simulink model "odev6_iremelmas_kara"  (R2023b)
settings: Solver=ode23tb  StartTime=0.0  StopTime=5  MaxStep=0.00001  RelTol=1e-5  EnableMultiTasking=on
libraries: spsSeriesRLCBranchLib x17, spsDiodeLib x2, spsThyristorLib x2, spsVoltageMeasurementLib x2, spsDCVoltageSourceLib x1, spsACVoltageSourceLib x1, powerlib_extras x1, spsCurrentMeasurementLib x1, spsDCMachineLib x1, spsFourierLib x1, spsMeanLib x1, spsRMSLib x1
settings Model: Creator=bb  LastModifiedBy=ireme
settings SolverCC: AlgebraicLoopSolver=TrustRegion
settings DataIOCC: SaveFormat=Array  SignalLoggingSaveFormat=ModelDataLogs  SaveOutput=off  SignalLogging=off  SaveTime=off  ReturnWorkspaceOutputs=off
settings OptimizationCC: ExpressionDepthLimit=2147483647  InitFltsAndDblsToZero=on  LifeSpan=inf
settings DebuggingCC: SaveWithParameterizedLinksMsg=none  UnderspecifiedInitializationDetection=Classic  MergeDetectMultiDrivingBlocksExec=none  SignalResolutionControl=TryResolveAllWithWarning  SolverPrmCheckMsg=warning  FcnCallInpInsideContextMsg=warning  UnconnectedInputMsg=warning  UnconnectedOutputMsg=warning  UnconnectedLineMsg=warning  StateNameClashWarn=warning  SFUnexpectedBacktrackingDiag=warning  SFNoUnconditionalDefaultTransitionDiag=warning  SFExecutionAtInitializationDiag=none  ArithmeticOperatorsInVariantConditions=warning
settings HardwareCC: ProdBitPerPointer=32  ProdBitPerSizeT=32  ProdBitPerPtrDiffT=32  ProdLargestAtomicFloat=None  ProdIntDivRoundTo=Undefined  ProdEndianess=Unspecified  ProdWordSize=32  ProdHWDeviceType=32-bit Generic
settings ModelReferenceCC: EnableRefExpFcnMdlSchedulingChecks=on  PropagateSignalLabelsOutOfModel=off
settings SFSimCC: SimUseLocalCustomCode=off  CustomCodeUndefinedFunction=UseInterfaceOnly
settings RTWCC: RTWUseLocalCustomCode=off
settings CodeAppCC: StateflowObjectComments=on
settings GRTTargetCC: TargetFcnLib=ansi_tfl_tmw.mat  TargetLangStandard=C89/C90 (ANSI)  CombineOutputUpdateFcns=off  GRTInterface=on
settings ConfigComp: CovMetricSettings=dw  CovSaveCumulativeToWorkspaceVar=on  CovSaveSingleToWorkspaceVar=on  CovExternalEMLEnable=off
settings SimscapeCC: SimscapeNormalizeSystem=off

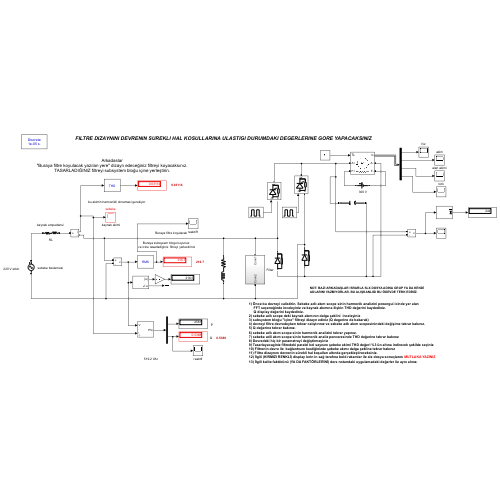
[thumbnail: Simulink's stored preview of the top-level diagram]
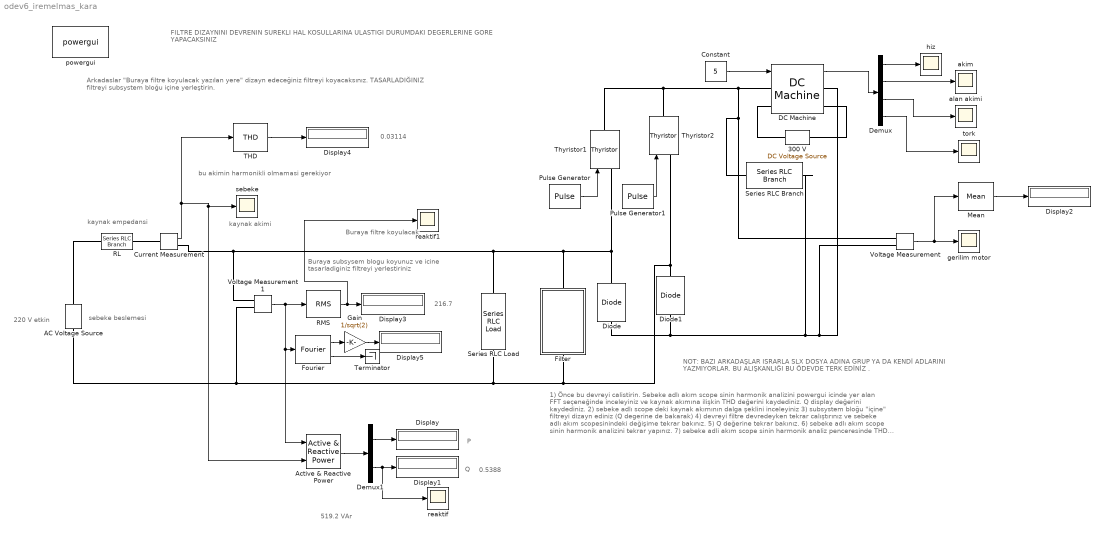
== system odev6_iremelmas_kara ==
  note: 220 V etkin
  note: NOT: BAZI ARKADAŞLAR ISRARLA SLX DOSYA ADINA GRUP YA DA KENDİ ADLARINI YAZMIYORLAR. BU ALIŞKANLIĞI BU ÖDEVDE TERK EDİNİZ .
  note: 216.7
  note: 0.5388
  note: 0.03114
  note: 519.2 VAr
  note: Q
  note: P
  note: Buraya filtre koyulacak
  note: Arkadaslar
      | "Buraya filtre koyulacak yazılan yere" dizayn edeceğiniz filtreyi koyacaksınız.
      | TASARLADIĞINIZ filtreyi subsystem bloğu içine yerleştirin.
  note: kaynak empedansi
  note: 1) Önce bu devreyi calistirin. Sebeke adlı akım scope sinin harmonik analizini powergui icinde yer alan
      | FFT seçeneğinde inceleyiniz ve kaynak akımına ilişkin THD değerini kaydediniz.
      | Q display değerini kaydediniz.
      | 2) sebeke adlı scope deki kaynak akımının dalga şeklini inceleyiniz
      | 3) subsystem bloğu "içine" filtreyi dizayn ediniz (Q degerine de bakarak)
      | 4) devreyi filtre devredeyken tekrar calıştırınız ve sebeke adlı akım scopesinindeki değişime tekrar bakınız.
      | 5) Q değerine tekrar bakınız.
      | 6) sebeke adlı akım scope sinin harmonik analizini tekrar yapınız.
      | 7) sebeke adli akım scope sinin harmonik analiz penceresinde THD değerine tekrar bakınız
      | 8) Devredeki hiç bir parametreyi değiştirmeyiniz
      | 9) Tasarlayacaginiz filtredeki paralel kol sayısını şebeke akimi THD değeri %3 ün altına indirecek şekilde seçiniz
      | 10) Filtrenin devre ile bağlantısını kestiğinizde şebeke akımı dalga şekline tekrar bakınız
      | 11) Filtre dizaynını devrenin sürekli hal koşulları altında gerçekleştireceksiniz.
      | 12) İlgili (KIRMIZI RENKLİ) display lerin in sağ tarafına bold rakamlar ile slx dosya sonuçlarını MUTLAKA YAZINIZ
      | 13) İlgili kalite faktörünü (YA DA FAKTÖRLERİNİ) ders notundaki uygulamadaki değerler ile aynı alınız.
  note: kaynak akimi
  note: bu akimin harmonikli olmamasi gerekiyor
  note: Buraya subsysem blogu koyunuz
      | ve icine tasarladiginiz  filtreyi yerlestiriniz
  note: sebeke beslemesi
  note: FILTRE DIZAYNINI DEVRENIN SUREKLI HAL KOSULLARINA ULASTIGI DURUMDAKI DEGERLERINE GORE YAPACAKSINIZ
  " 300 V" : spsDCVoltageSourceLib/DC Voltage Source  Amplitude=300  Measurements=None
  AC Voltage Source : spsACVoltageSourceLib/AC Voltage Source  Amplitude=220*sqrt(2)  Phase=0  Frequency=50  SampleTime=0  Measurements=None  BusType=swing  Pref=10e3  Qref=0  Qmin=-inf  Qmax=+inf
  Active & Reactive Power : powerlib_extras/Measurements/Active & Reactive Power  f1=50
  Constant : Constant  Value=5
  Current Measurement : spsCurrentMeasurementLib/Current Measurement  PhasorSimulation=off  OutputType=Complex  PSBequivalent=0
  DC Machine : spsDCMachineLib/DC Machine  PresetModel=01: 5HP 240V 1750RPM Field:300V  MechanicalLoad=Torque TL  FieldType=Wound  ShowDetailedParameters=on  MeasurementBus=off  RLa=[2.581 0.028]  RLf=[281.2 156]  Laf=0.9483  MachineConstant=Torque constant (N.m/A)  Ke=1.8  Kt=1.8  J=0.02215  Bm=0.002953  Tf=0.5161  w0=0  Ifinit=1.06685632871799  TsPowergui=0  TsBlock=-1
  Demux : Demux
  Demux1 : Demux  Outputs=2
  Diode : spsDiodeLib/Diode  Ron=0.001  Lon=0  Vf=0.8  IC=0  UseSnubber=off  Rs=500  Cs=250e-9  Measurements=off
  Diode1 : spsDiodeLib/Diode  Ron=0.001  Lon=0  Vf=0.8  IC=0  UseSnubber=off  Rs=500  Cs=250e-9  Measurements=off
  Display{,1..5} (6 alike) : Display
  Filter : Subsystem
  Fourier : spsFourierLib/Fourier  Freq=50  n=1  InInit=[0, 0]  Ts=0
  Gain : Gain  Gain=1/sqrt(2)
  Mean : spsMeanLib/Mean  Freq=50  Vinit=0  Ts=0
  Pulse Generator : DiscretePulseGenerator  PulseType=Time based  Period=0.02  PulseWidth=15  PhaseDelay=0.66*0.01
  Pulse Generator1 : DiscretePulseGenerator  PulseType=Time based  Period=0.02  PulseWidth=15  PhaseDelay=0.66*0.01+0.01
  RL : spsSeriesRLCBranchLib/Series RLC Branch  LConnTagsString=__new0  RConnTagsString=__new0  BranchType=RL  Resistance=0.2  Inductance=6e-3  SetiL0=off  InitialCurrent=0  Capacitance=1e-6  Setx0=off  InitialVoltage=0  Measurements=None
  RMS : spsRMSLib/RMS  TrueRMS=on  Freq=50  RMSInit=100  Ts=0
  Series RLC Branch : spsSeriesRLCBranchLib/Series RLC Branch  LConnTagsString=__new0  RConnTagsString=__new0  BranchType=C  Resistance=1  Inductance=1e-3  SetiL0=off  InitialCurrent=0  Capacitance=2e-1  Setx0=off  InitialVoltage=0  Measurements=None
  Series RLC Load : spsSeriesRLCLoadLib/Series RLC Load  LConnTagsString=a  RConnTagsString=__new0  NominalVoltage=220  NominalFrequency=50  ActivePower=10e2  InductivePower=10000  CapacitivePower=0  Setx0=off  InitialVoltage=0  SetiL0=off  InitialCurrent=0  Measurements=None  LoadType=constant Z
  THD : spsTHDLib/THD  Freq=50  Ts=0
  Terminator : Terminator
  Thyristor1 : spsThyristorLib/Thyristor  Ron=1e-3  Lon=0  Vf=0.8  IC=0  Rs=200  Cs=4e-6  Measurements=off
      settings: AttributesFormatString=\n
  Thyristor2 : spsThyristorLib/Thyristor  Ron=1e-3  Lon=0  Vf=0.8  IC=0  Rs=200  Cs=4e-6  Measurements=off
      settings: AttributesFormatString=\n
  Voltage Measurement : spsVoltageMeasurementLib/Voltage Measurement  PhasorSimulation=off  OutputType=Complex  PSBequivalent=0
  Voltage Measurement1 : spsVoltageMeasurementLib/Voltage Measurement  PhasorSimulation=off  OutputType=Complex  PSBequivalent=0
  akim : Scope
  alan akimi : Scope
  gerilim motor : Scope
  hiz : Scope
  powergui : spspowerguiLib/powergui  SimulationMode=Discrete  SampleTime=1e-5  frequency=50  Iterations=50  frequencyindice=0  Pbase=100e6  ErrMax=1e-4  UnitsV=kV  UnitsW=MW  buscounter=0  FunctionMessages=off  echomessages=off  EnableUseOfTLC=off  CurrentSourceSwitches=off  DisableSnubberDevices=off  DisableRonSwitches=off  DisableVfSwitches=off  DisplayEquations=off  AutomaticDiscreteSolvers=off  SolverType=Tustin  Interpol=off  ExternalGateDelay=off  methode=off  Ts=0  x0status=steady  SPID=off  SwTol=0  HookPort=off  NonlinearTolerance=1e-4  nMaxIteration=100  ContinueOnMaxIteration=off  RestoreLinks=warning  ResistiveCurrentMeasurement=off  Frange=[0:2:500]  Ylog=off  Xlog=on  ShowGrid=off  save=off  variable=ZData  structure=sebeke  ZoomFFT=off  StartTime=1.6  cycles=4  DisplayStyle=4  fundamental=50  FreqAxis=off  MaxFrequency=1000  frequencyindicesteady=1  RmsSteady=1  display=off
  reaktif : Scope
  reaktif1 : Scope
  sebeke : Scope
  tork : Scope
  wires:
  Constant/1 -> DC Machine/1
  DC Machine/1 -> Demux/1
  Demux/1 -> hiz/1
  Demux/2 -> akim/1
  Demux/3 -> alan akimi/1
  Demux/4 -> tork/1
  Current Measurement/1 -> THD/1, Active & Reactive Power/2, sebeke/1
  Voltage Measurement1/1 -> RMS/1, Fourier/1, Active & Reactive Power/1
  Active & Reactive Power/1 -> Demux1/1
  Demux1/1 -> Display/1
  Demux1/2 -> Display1/1, reaktif/1
  Voltage Measurement/1 -> Mean/1, gerilim motor/1
  Mean/1 -> Display2/1
  RMS/1 -> reaktif1/1, Display3/1
  THD/1 -> Display4/1
  Fourier/2 -> Terminator/1
  Fourier/1 -> Gain/1
  Gain/1 -> Display5/1
  Pulse Generator1/1 -> Thyristor2/1
  Pulse Generator/1 -> Thyristor1/1
  connections:
  " 300 V"/RConn1 -- DC Machine/LConn2
  " 300 V"/LConn1 -- DC Machine/RConn2
  Series RLC Branch/LConn1 -- Voltage Measurement/LConn1 -- Thyristor2/RConn1 -- Thyristor1/RConn1 -- DC Machine/LConn1
  Current Measurement/RConn1 -- Series RLC Load/LConn1 -- Filter/RConn1 -- Diode/RConn1 -- Thyristor1/LConn1 -- Voltage Measurement1/LConn1
  AC Voltage Source/LConn1 -- Filter/LConn1 -- Thyristor2/LConn1 -- Diode1/RConn1 -- Series RLC Load/RConn1 -- Voltage Measurement1/LConn2
  DC Machine/RConn1 -- Voltage Measurement/LConn2 -- Series RLC Branch/RConn1 -- Diode/LConn1 -- Diode1/LConn1
  AC Voltage Source/RConn1 -- RL/LConn1
  RL/RConn1 -- Current Measurement/LConn1

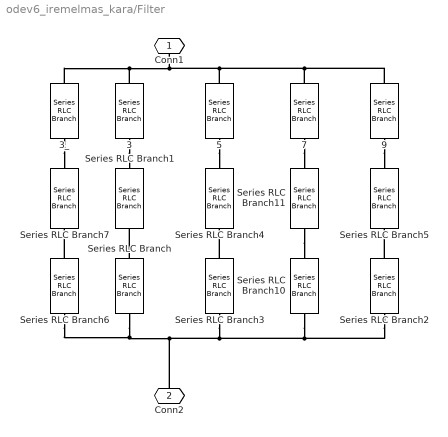
== system odev6_iremelmas_kara/Filter ==
  {3,5,7,9} (4 alike) : spsSeriesRLCBranchLib/Series RLC Branch  LConnTagsString=__new0  RConnTagsString=__new0  BranchType=C  Resistance=1  Inductance=1e-3  SetiL0=off  InitialCurrent=0  Capacitance=0.00013674  Setx0=off  InitialVoltage=0  Measurements=None
  3_ : spsSeriesRLCBranchLib/Series RLC Branch  LConnTagsString=__new0  RConnTagsString=__new0  BranchType=C  Resistance=1  Inductance=1e-3  SetiL0=off  InitialCurrent=0  Capacitance=0.00013674  Setx0=off  InitialVoltage=0  Measurements=None
  Series RLC Branch : spsSeriesRLCBranchLib/Series RLC Branch  LConnTagsString=__new0  RConnTagsString=__new0  BranchType=R  Resistance=0.2217  Inductance=1e-3  SetiL0=off  InitialCurrent=0  Capacitance=1e-6  Setx0=off  InitialVoltage=0  Measurements=None
  Series RLC Branch1 : spsSeriesRLCBranchLib/Series RLC Branch  LConnTagsString=__new0  RConnTagsString=__new0  BranchType=L  Resistance=1  Inductance=0.0082332  SetiL0=off  InitialCurrent=0  Capacitance=1e-6  Setx0=off  InitialVoltage=0  Measurements=None
  Series RLC Branch10 : spsSeriesRLCBranchLib/Series RLC Branch  LConnTagsString=__new0  RConnTagsString=__new0  BranchType=R  Resistance=0.095016  Inductance=1e-3  SetiL0=off  InitialCurrent=0  Capacitance=1e-6  Setx0=off  InitialVoltage=0  Measurements=None
  Series RLC Branch11 : spsSeriesRLCBranchLib/Series RLC Branch  LConnTagsString=__new0  RConnTagsString=__new0  BranchType=L  Resistance=1  Inductance=0.0015122  SetiL0=off  InitialCurrent=0  Capacitance=1e-6  Setx0=off  InitialVoltage=0  Measurements=None
  Series RLC Branch2 : spsSeriesRLCBranchLib/Series RLC Branch  LConnTagsString=__new0  RConnTagsString=__new0  BranchType=R  Resistance=0.073901  Inductance=1e-3  SetiL0=off  InitialCurrent=0  Capacitance=1e-6  Setx0=off  InitialVoltage=0  Measurements=None
  Series RLC Branch3 : spsSeriesRLCBranchLib/Series RLC Branch  LConnTagsString=__new0  RConnTagsString=__new0  BranchType=R  Resistance=0.13302  Inductance=1e-3  SetiL0=off  InitialCurrent=0  Capacitance=1e-6  Setx0=off  InitialVoltage=0  Measurements=None
  Series RLC Branch4 : spsSeriesRLCBranchLib/Series RLC Branch  LConnTagsString=__new0  RConnTagsString=__new0  BranchType=L  Resistance=1  Inductance=0.002964  SetiL0=off  InitialCurrent=0  Capacitance=1e-6  Setx0=off  InitialVoltage=0  Measurements=None
  Series RLC Branch5 : spsSeriesRLCBranchLib/Series RLC Branch  LConnTagsString=__new0  RConnTagsString=__new0  BranchType=L  Resistance=1  Inductance=0.0009148  SetiL0=off  InitialCurrent=0  Capacitance=1e-6  Setx0=off  InitialVoltage=0  Measurements=None
  Series RLC Branch6 : spsSeriesRLCBranchLib/Series RLC Branch  LConnTagsString=__new0  RConnTagsString=__new0  BranchType=R  Resistance=0.2217  Inductance=1e-3  SetiL0=off  InitialCurrent=0  Capacitance=1e-6  Setx0=off  InitialVoltage=0  Measurements=None
  Series RLC Branch7 : spsSeriesRLCBranchLib/Series RLC Branch  LConnTagsString=__new0  RConnTagsString=__new0  BranchType=L  Resistance=1  Inductance=0.0082332  SetiL0=off  InitialCurrent=0  Capacitance=1e-6  Setx0=off  InitialVoltage=0  Measurements=None
  Conn1 : PMIOPort  Side=Right
  Conn2 : PMIOPort  Port=2  Side=Left
  connections:
  7/RConn1 -- Series RLC Branch11/LConn1
  Series RLC Branch3/LConn1 -- Series RLC Branch4/RConn1
  5/RConn1 -- Series RLC Branch4/LConn1
  Series RLC Branch/LConn1 -- Series RLC Branch1/RConn1
  3/RConn1 -- Series RLC Branch1/LConn1
  Series RLC Branch11/RConn1 -- Series RLC Branch10/LConn1
  9/RConn1 -- Series RLC Branch5/LConn1
  Series RLC Branch2/LConn1 -- Series RLC Branch5/RConn1
  9/LConn1 -- 7/LConn1 -- 5/LConn1 -- 3_/LConn1 -- 3/LConn1 -- Conn1/RConn1
  Conn2/RConn1 -- Series RLC Branch6/RConn1 -- Series RLC Branch/RConn1 -- Series RLC Branch2/RConn1 -- Series RLC Branch10/RConn1 -- Series RLC Branch3/RConn1
  3_/RConn1 -- Series RLC Branch7/LConn1
  Series RLC Branch6/LConn1 -- Series RLC Branch7/RConn1
